simulink model "mountain_uav_unreal"  (R2025b)
settings: Solver=VariableStepAuto  StartTime=0.0  StopTime=8  RelTol=1e-3
libraries: sim3dautolib x3, sim3dcameralib x1, uavsim3dlib x1, sim3dlib x1
settings Model: Creator=lab  LastModifiedBy=lab

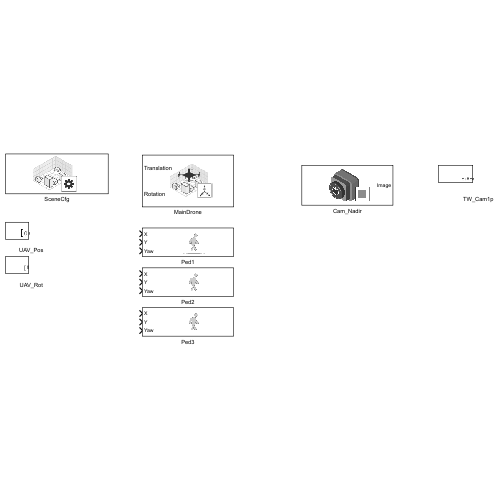
[thumbnail: Simulink's stored preview of the top-level diagram]
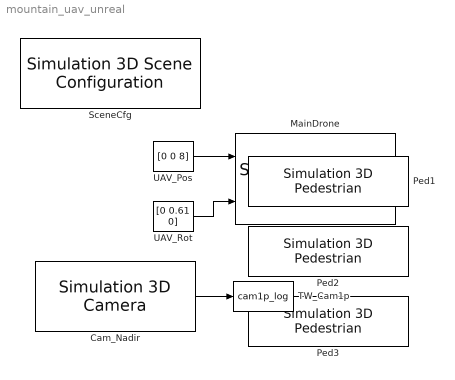
== system mountain_uav_unreal ==
  Cam_Nadir : sim3dcameralib/Simulation 3D Camera  Priority=1  sensorTag=Sim3dSensor  sensorId=1  sensorName=Sim3dSensor  vehTagList={'Scene Origin', 'MainDrone'}  vehTag=MainDrone  CoordinateSystem=ISO8855  mountLoc=Origin  offsetFlag=on  tmountOffset=[0 0 0]  extTmount=off  rmountOffset=[0 0 0]  extRmount=off  FocalLength=[1109, 1109]  OpticalCenter=[640, 360]  ImageSize=[640 360]  RadialDistortion=[0, 0]  TangentialDistortion=[0, 0]  SensorSkew=0  VisualizeFieldOfView=off  FieldOfViewRange=61  DepthOutportEnabled=off  SemanticOutportEnabled=off  TransformOutportEnabled=off  SampleTime=0.1  mountPoint=[0 0 0]  mountOrientation=[0 0 0]  aMode=4  ID=1
      settings: LibrarySourceBlock=uavsim3dlib/Simulation 3D Camera
  MainDrone : uavsim3dlib/Simulation 3D UAV Vehicle  Priority=-1  Mesh=Quadrotor  MeshPath=/MathWorksUAVContent/UAVs/HexaRotorUAV/HexaRotor.HexaRotor  Color=Red  ActorName=MainDrone  UseGlobalFrame=off  InitialTranslation=[0 0 8]  InitialRotation=[0 0.61 0]  InitialTranslationGlobal=[0 0 0]  InitialGeoOrigin=[0 0 0]  InitialRotationGlobal=[0 0 0]  SampleTime=0.05  ActorType=SimulinkVehicle  ID=C  aMode=4  ActorTag=MainDrone
  Ped1 : sim3dautolib/Simulation 3D Pedestrian  Priority=-1  PedestrianType=Male 1  Scale=[1, 1, 1]  CoordinateSystem=ISO8855  InitialPos=[10 -1 0]  InitialYaw=0  ActorName=SimulinkPedestrian1  SampleTime=-1  ActorType=SimulinkPedestrian  ActorTag=SimulinkPedestrian1  ID=1  aMode=3  CoordinateScheme=0  TransformOutportEnabled=off
      settings: LibrarySourceBlock=drivingsim3d/Simulation 3D Pedestrian
  Ped2 : sim3dautolib/Simulation 3D Pedestrian  Priority=-1  PedestrianType=Female 2  Scale=[1, 1, 1]  CoordinateSystem=ISO8855  InitialPos=[11 1 0]  InitialYaw=90  ActorName=SimulinkPedestrian2  SampleTime=-1  ActorType=SimulinkPedestrian  ActorTag=SimulinkPedestrian2  ID=2  aMode=3  CoordinateScheme=0  TransformOutportEnabled=off
      settings: LibrarySourceBlock=drivingsim3d/Simulation 3D Pedestrian
  Ped3 : sim3dautolib/Simulation 3D Pedestrian  Priority=-1  PedestrianType=Male 2  Scale=[1, 1, 1]  CoordinateSystem=ISO8855  InitialPos=[13 -2 0]  InitialYaw=180  ActorName=SimulinkPedestrian3  SampleTime=-1  ActorType=SimulinkPedestrian  ActorTag=SimulinkPedestrian3  ID=3  aMode=3  CoordinateScheme=0  TransformOutportEnabled=off
      settings: LibrarySourceBlock=drivingsim3d/Simulation 3D Pedestrian
  SceneCfg : sim3dlib/Simulation 3D Scene Configuration  Priority=0  ProjectFormat=Default Scenes  SceneDesc=Empty Grass  ProjectName=C:\Program Files\MATLAB\R2025b\toolbox\shared\sim3d_projects\automotive_project_windows\UE\WindowsNoEditor\VehicleSimulation.exe  ScenePath=/Game/Maps/USCityBlock  EnableOpenDRIVE=off  vehTagList={'Custom';'Scene Origin'}  vehTag=Scene Origin  AttachedCameraRelativeTranslation=[0 0 0]  FreeCameraDefaultInitialTranslation=[-6, 0, 2]  AttachedCameraRelativeRotation=[0 0 0]  FreeCameraDefaultInitialRotation=[0, -15, 0]  ViewpointName=Custom  FreeCameraInitialTranslation=[-15 0 12]  ViewpointTranslation=[0, 0, 0]  FreeCameraInitialRotation=[0 0.30 0]  ViewpointRotation=[0, 0, 0]  OpVisEn=off  Ts=0.05  EnableWindow=on  EnableRemoteAccess=off  EnableWeather=on  SunAzimuth=180  SunAltitude=60  EnableGeospatialSun=off  Latitude=0  Longitude=0  Date=2023-01-01  Time=10:30:00  GeoTimeZone=-5.0  SunDaylightSaving=off  wind=1  clouds=10  EnableVolumetricClouds=off  CloudCoverage=0  CloudAltitude=6  fog=0  rain=0  RaindropsEffect=off  SnowDensity=0  EnableGeospatial=off  TilesetSource=Earth terrain  UseTrueOrigin=off  OriginHeight=200  OriginLatitude=40.744652  OriginLongitude=-73.988864  MapStyle=Aerial  AdditionalAssetIDs=[]  UseAdvancedSunSky=off  SolarTime=11  TimeZone=-5  Day=21  Month=9  Year=2022  UseDaylightSavingTime=on  DSTStartDay=10  DSTStartMonth=3  DSTEndDay=3  DSTEndMonth=11  DSTSwitchHour=2  sensorTag=MainCamera1  sensorId=1  sensorName=MainCamera1  mountLoc=Origin  offsetFlag=off  tmountOffset=[0, 0, 0]  rmountOffset=[0, 0, 0]  HorizontalResolution=1280  VerticalResolution=720  HorizontalFOV=60  mountPoint=[0 0 0]  mountOrientation=[0 0 0]  aMode=4  ID=1  GeoTrigger=Inactive  ViewNameList={'Custom'}  ViewTranslationList={'[-15 0 12]'}  ViewRotationList={'[0 0.3 0]'}
      settings: LibrarySourceBlock=uavsim3dlib/Simulation 3D Scene Configuration
  TW_Cam1p : ToWorkspace  VariableName=cam1p_log  SaveFormat=Structure With Time  SampleTime=0.1
  UAV_Pos : Constant  Value=[0 0 8]
  UAV_Rot : Constant  Value=[0 0.61 0]
  wires:
  UAV_Rot/1 -> MainDrone/2
  UAV_Pos/1 -> MainDrone/1
  Cam_Nadir/1 -> TW_Cam1p/1
